simulink model "statefeedbackcontroledsystem"  (R2018b)
settings: Solver=VariableStepAuto  StartTime=0.0  StopTime=40  RelTol=1e-3
settings Model: Creator=ASUS  LastModifiedBy=ASUS

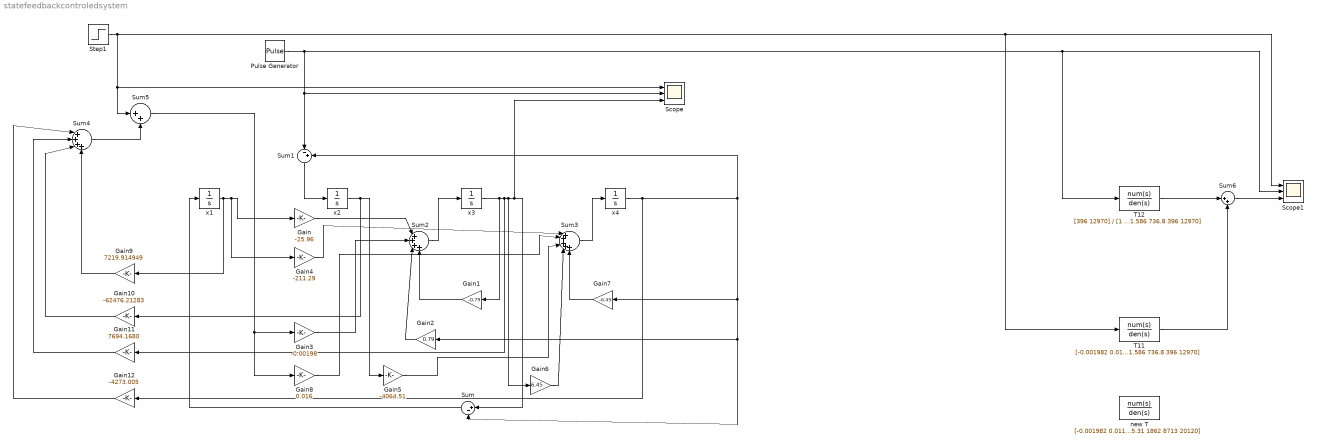
== system statefeedbackcontroledsystem ==
  Gain : Gain  Gain=-25.96
  Gain1 : Gain  Gain=-0.79
  Gain10 : Gain  Gain=-62476.21283
  Gain11 : Gain  Gain=7694.1680
  Gain12 : Gain  Gain=-4273.005
  Gain2 : Gain  Gain=0.79
  Gain3 : Gain  Gain=-0.00198
  Gain4 : Gain  Gain=-211.29
  Gain5 : Gain  Gain=-4064.51
  Gain6 : Gain  Gain=6.45
  Gain7 : Gain  Gain=-6.45
  Gain8 : Gain  Gain=0.016
  Gain9 : Gain  Gain=7219.914949
  Pulse Generator : DiscretePulseGenerator  PulseType=Time based  Period=30  PulseWidth=10  PhaseDelay=5
  Scope : Scope  NumInputPorts=3
  Scope1 : Scope  NumInputPorts=3
  Step1 : Step  SampleTime=0
  Sum : Sum  Inputs=|+-
  Sum1 : Sum  Inputs=|-+
  Sum2 : Sum  Inputs=|++++
  Sum3 : Sum  Inputs=|+++++
  Sum4 : Sum  Inputs=|++++
  Sum5 : Sum  Inputs=|++
  Sum6 : Sum  Inputs=|++
  T11 : TransferFcn  Numerator=[-0.001982 0.01122 -0.9901 0]  Denominator=[1 1.586 736.8 396 12970]
  T12 : TransferFcn  Numerator=[396 12970]  Denominator=[1 1.586 736.8 396 12970]
  new T : TransferFcn  Numerator=[-0.001982 0.01122 -0.9901 0]  Denominator=[1 85.31 1862 8713 20120]
  x{1..4} (4 alike) : Integrator
  wires:
  Gain3/1 -> Sum2/2
  Gain2/1 -> Sum2/3
  Gain7/1 -> Sum3/5
  Gain1/1 -> Sum2/4
  Gain6/1 -> Sum3/4
  Gain/1 -> Sum2/1
  Sum2/1 -> x3/1
  Sum5/1 -> Gain8/1, Gain3/1
  Gain4/1 -> Sum3/1
  Gain8/1 -> Sum3/2
  Sum/1 -> x1/1
  x1/1 -> Gain9/1, Gain4/1, Gain/1
  Sum1/1 -> x2/1
  Sum3/1 -> x4/1
  Pulse Generator/1 -> Sum1/1, Scope/2, Scope1/2, T12/1
  x3/1 -> Gain11/1, Gain6/1, Scope/3, Sum/1, Gain1/1
  x4/1 -> Gain12/1, Sum1/2, Gain7/1, Gain2/1, Sum/2
  x2/1 -> Gain10/1, Gain5/1
  Gain5/1 -> Sum3/3
  Gain9/1 -> Sum4/4
  Gain10/1 -> Sum4/3
  Gain11/1 -> Sum4/2
  Gain12/1 -> Sum4/1
  Sum4/1 -> Sum5/2
  Step1/1 -> Scope1/1, T11/1, Sum5/1, Scope/1
  T12/1 -> Sum6/1
  T11/1 -> Sum6/2
  Sum6/1 -> Scope1/3
